simulink model "Scheme"  (R2014a)
settings: Solver=ode45  SolverMode=SingleTasking  StartTime=0.0  StopTime=5.0  RelTol=1e-3
libraries: commsink2 x1, dspsigops x1, simulink x1, dspsrcs4 x1
settings Model: Creator=Olia  LastModifiedBy=olia-PC
settings OptimizationCC: BlockReduction=off  BooleanDataType=off  SimCompilerOptimization=off
settings DebuggingCC: SaveWithParameterizedLinksMsg=none  UnderspecifiedInitializationDetection=Classic  SignalResolutionControl=TryResolveAllWithWarning  SolverPrmCheckMsg=none  FrameProcessingCompatibilityMsg=error  StrictBusMsg=Warning
settings HardwareCC: TargetUnknown=on
settings RTWCC: RTWCompilerOptimization=off

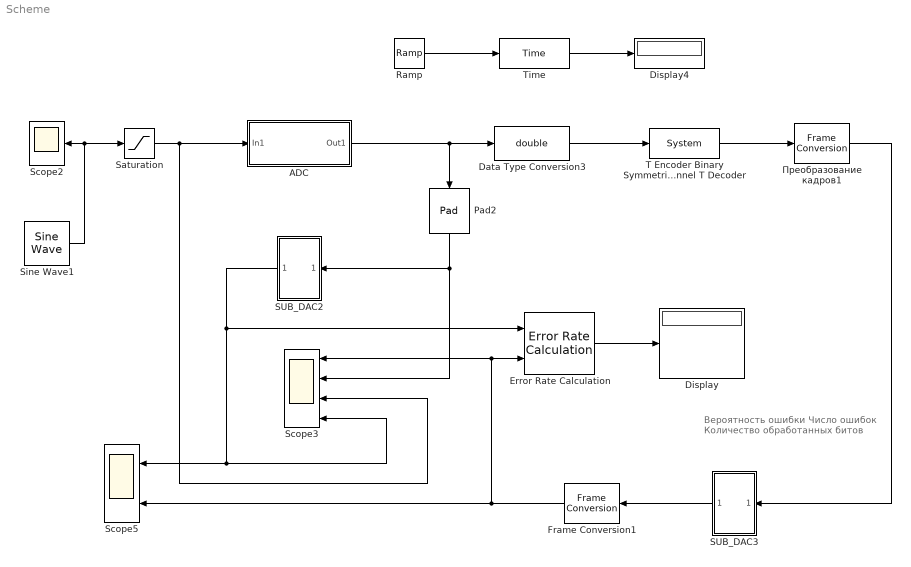
== system Scheme ==
  note: Вероятность ошибки
      | Число ошибок
      | Количество обработанных битов
  ADC : Subsystem
  Data Type Conversion3 : DataTypeConversion  OutDataTypeStr=double
  Display : Display
  Display4 : Display
  Error Rate Calculation : commsink2/Error Rate Calculation  N=0  st_delay=0  cp_mode=Entire frame  subframe=[]  PMode=Port  WsName=ErrorVec1  RsMode2=off  stop=off  numErr=maxNumErrs  maxBits=maxNumBits
  Frame Conversion1 : FrameConversion  OutFrame=Sample-based
  Pad2 : dspsigops/Pad  padAlong=Columns  dimsToPad=1  valSrc=Specify via dialog  padVal=1  spec=Output size  padNumOutRowsSpecMethod=User-specified  numOutRows=16  padNumOutColsSpecMethod=User-specified  numOutCols=1  isVarDimsMode=off  padBeginning=0  padEnd=0  outSizeMode=User-specified  outSize=1  padSigAt=Beginning  trunc_flag=None  roundingMode=Floor  overflowMode=off  truncOrWrapMode=Truncate  wrap_flag=None
  Ramp : simulink/Sources/Ramp  slope=1  start=0  X0=0
  SUB_DAC2 : Subsystem
  SUB_DAC3 : Subsystem
  Saturation : Saturate  UpperLimit=2^24-1  LowerLimit=0
  Scope2 : Scope
      settings: TickLabels=on  YMin=0  YMax=10  SaveName=ScopeData2
  Scope3 : Scope  NumInputPorts=4
      settings: TickLabels=on  TimeRange=3  YMin=0~-5~-5~-5  YMax=3~10~10~5  SaveName=ScopeData5
  Scope5 : Scope  NumInputPorts=2
      settings: TickLabels=on  YMin=0~0  YMax=3~6e-06  SaveName=ScopeData4
  Sine Wave1 : dspsrcs4/Sine Wave  Amplitude=10  Frequency=2  Phase=0  SampleMode=Discrete  OutComplex=Real  CompMethod=Trigonometric fcn  TableSize=Speed  SampleTime=1/70  SamplesPerFrame=1  ResetState=Restart at time zero  dataType=double  wordLen=16  udDataType=sfix(16)  fracBitsMode=Best precision  numFracBits=15  OutDataTypeStr=double  LastOutDataTypeStr=double
  T Encoder Binary Symmetric Channel T Decoder : MATLABFcn  MATLABFcn=System
  Time : MATLABFcn  MATLABFcn=Time
  Преобразование кадров1 : FrameConversion
  wires:
  Error Rate Calculation/1 -> Display/1
  Sine Wave1/1 -> Scope2/1, Saturation/1
  Saturation/1 -> Scope3/3, ADC/1(In1)
  SUB_DAC3/1(Out1) -> Frame Conversion1/1
  Frame Conversion1/1 -> Scope5/2, Scope3/1, Error Rate Calculation/2
  SUB_DAC2/1(Out1) -> Scope3/4, Scope5/1, Error Rate Calculation/1
  ADC/1(Out1) -> Pad2/1, Data Type Conversion3/1
  Преобразование кадров1/1 -> SUB_DAC3/1(In2)
  Pad2/1 -> Scope3/2, SUB_DAC2/1(In2)
  Time/1 -> Display4/1
  Ramp/1 -> Time/1
  Data Type Conversion3/1 -> T Encoder Binary Symmetric Channel T Decoder/1
  T Encoder Binary Symmetric Channel T Decoder/1 -> Преобразование кадров1/1

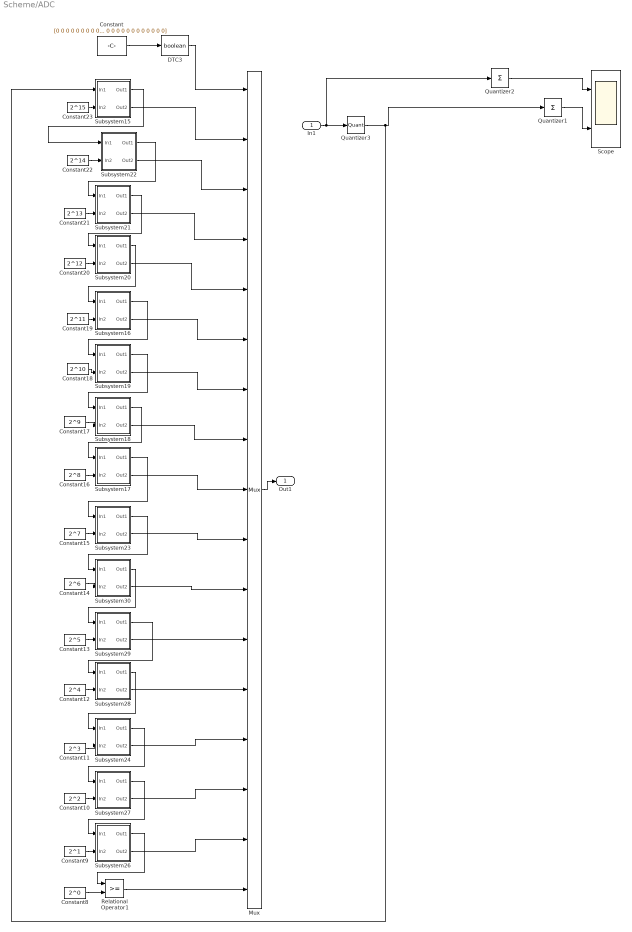
== system Scheme/ADC ==
  In1 : Inport
  Constant : Constant  Value=[0 0 0 0 0 0 0 0 0 0 0 0 0 0 0 0 0 0 0 0 0 0 0 0 0 0 0 0 0 0 0 0 0 0 0 0 0 0 0 0 0 0 0 0 0 0 0 0 0 0 0 0 0 0 0]
  Constant10 : Constant  Value=2^2
  Constant11 : Constant  Value=2^3
  Constant12 : Constant  Value=2^4
  Constant13 : Constant  Value=2^5
  Constant14 : Constant  Value=2^6
  Constant15 : Constant  Value=2^7
  Constant16 : Constant  Value=2^8
  Constant17 : Constant  Value=2^9
  Constant18 : Constant  Value=2^10
  Constant19 : Constant  Value=2^11
  Constant20 : Constant  Value=2^12
  Constant21 : Constant  Value=2^13
  Constant22 : Constant  Value=2^14
  Constant23 : Constant  Value=2^15
  Constant8 : Constant  Value=2^0
  Constant9 : Constant  Value=2^1
  DTC3 : DataTypeConversion  OutDataTypeStr=boolean  LockScale=on
  Mux : Mux  Inputs=17
  Quantizer1 : Sum  Inputs=+
  Quantizer2 : Sum  Inputs=+
  Quantizer3 : Quantizer  QuantizationInterval=0.2
  Relational Operator1 : RelationalOperator  OutDataTypeStr=boolean
  Scope : Scope  NumInputPorts=2
      settings: YMin=-5~-5  YMax=5~5
  Subsystem15 : Subsystem
  Subsystem16 : Subsystem
  Subsystem17 : Subsystem
  Subsystem18 : Subsystem
  Subsystem19 : Subsystem
  Subsystem20 : Subsystem
  Subsystem21 : Subsystem
  Subsystem22 : Subsystem
  Subsystem23 : Subsystem
  Subsystem24 : Subsystem
  Subsystem26 : Subsystem
  Subsystem27 : Subsystem
  Subsystem28 : Subsystem
  Subsystem29 : Subsystem
  Subsystem30 : Subsystem
  Out1 : Outport
  wires:
  Subsystem15/1(Out1) -> Subsystem22/1(In1)
  Quantizer3/1 -> Quantizer1/1, Subsystem15/1(In1)
  Quantizer1/1 -> Scope/2
  Quantizer2/1 -> Scope/1
  Mux/1 -> Out1/1
  In1/1 -> Quantizer2/1, Quantizer3/1
  Subsystem28/1(Out1) -> Subsystem24/1(In1)
  Constant11/1 -> Subsystem24/2(In2)
  Subsystem20/1(Out1) -> Subsystem16/1(In1)
  Subsystem17/1(Out1) -> Subsystem23/1(In1)
  Subsystem26/1(Out1) -> Relational Operator1/1
  Subsystem29/1(Out1) -> Subsystem28/1(In1)
  Subsystem18/1(Out1) -> Subsystem17/1(In1)
  Subsystem21/1(Out1) -> Subsystem20/1(In1)
  Constant22/1 -> Subsystem22/2(In2)
  Constant21/1 -> Subsystem21/2(In2)
  Constant19/1 -> Subsystem16/2(In2)
  Constant20/1 -> Subsystem20/2(In2)
  Constant9/1 -> Subsystem26/2(In2)
  Constant10/1 -> Subsystem27/2(In2)
  Constant12/1 -> Subsystem28/2(In2)
  Constant13/1 -> Subsystem29/2(In2)
  Constant14/1 -> Subsystem30/2(In2)
  Constant15/1 -> Subsystem23/2(In2)
  Constant16/1 -> Subsystem17/2(In2)
  Constant17/1 -> Subsystem18/2(In2)
  Constant18/1 -> Subsystem19/2(In2)
  Constant23/1 -> Subsystem15/2(In2)
  Constant8/1 -> Relational Operator1/2
  Subsystem27/1(Out1) -> Subsystem26/1(In1)
  Subsystem24/1(Out1) -> Subsystem27/1(In1)
  Subsystem30/1(Out1) -> Subsystem29/1(In1)
  Subsystem23/1(Out1) -> Subsystem30/1(In1)
  Subsystem19/1(Out1) -> Subsystem18/1(In1)
  Subsystem16/1(Out1) -> Subsystem19/1(In1)
  Subsystem22/1(Out1) -> Subsystem21/1(In1)
  Relational Operator1/1 -> Mux/17
  Subsystem26/2(Out2) -> Mux/16
  Subsystem27/2(Out2) -> Mux/15
  Subsystem24/2(Out2) -> Mux/14
  Subsystem28/2(Out2) -> Mux/13
  Subsystem29/2(Out2) -> Mux/12
  Subsystem30/2(Out2) -> Mux/11
  Subsystem23/2(Out2) -> Mux/10
  Subsystem17/2(Out2) -> Mux/9
  Subsystem18/2(Out2) -> Mux/8
  Subsystem19/2(Out2) -> Mux/7
  Subsystem16/2(Out2) -> Mux/6
  Subsystem20/2(Out2) -> Mux/5
  Subsystem21/2(Out2) -> Mux/4
  Subsystem22/2(Out2) -> Mux/3
  Subsystem15/2(Out2) -> Mux/2
  Constant/1 -> DTC3/1
  DTC3/1 -> Mux/1

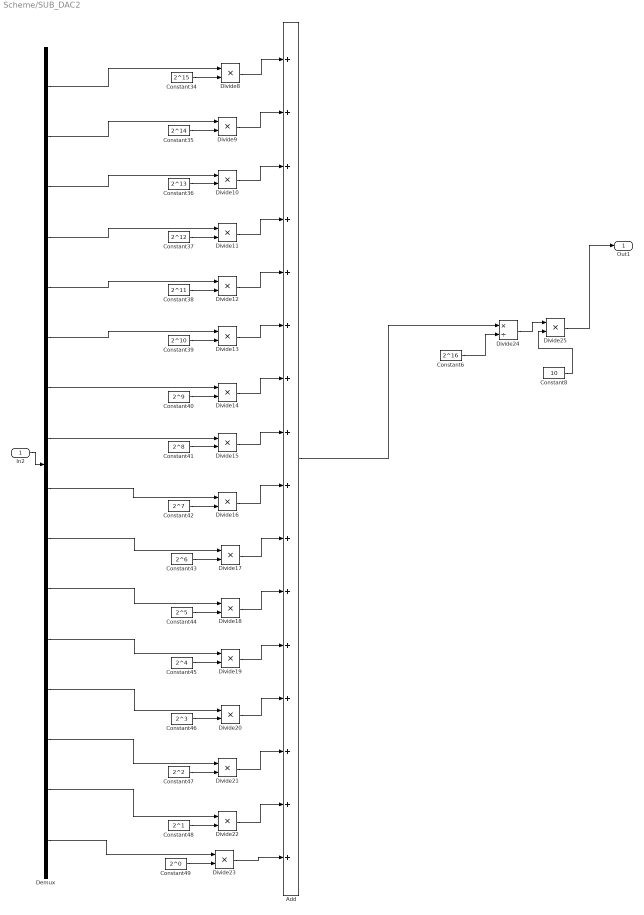
== system Scheme/SUB_DAC2 ==
  In2 : Inport
  Add : Sum  Inputs=++++++++++++++++
  Constant34 : Constant  Value=2^15
  Constant35 : Constant  Value=2^14
  Constant36 : Constant  Value=2^13
  Constant37 : Constant  Value=2^12
  Constant38 : Constant  Value=2^11
  Constant39 : Constant  Value=2^10
  Constant40 : Constant  Value=2^9
  Constant41 : Constant  Value=2^8
  Constant42 : Constant  Value=2^7
  Constant43 : Constant  Value=2^6
  Constant44 : Constant  Value=2^5
  Constant45 : Constant  Value=2^4
  Constant46 : Constant  Value=2^3
  Constant47 : Constant  Value=2^2
  Constant48 : Constant  Value=2^1
  Constant49 : Constant  Value=2^0
  Constant6 : Constant  Value=2^16
  Constant8 : Constant  Value=10
  Demux : Demux  Outputs=16
  Divide{8..23,25} (17 alike) : Product  Inputs=**
  Divide24 : Product  Inputs=*/
  Out1 : Outport
  wires:
  Constant49/1 -> Divide23/2
  Constant48/1 -> Divide22/2
  Constant47/1 -> Divide21/2
  Constant46/1 -> Divide20/2
  Constant45/1 -> Divide19/2
  Constant44/1 -> Divide18/2
  Constant43/1 -> Divide17/2
  Constant42/1 -> Divide16/2
  Constant41/1 -> Divide15/2
  Constant40/1 -> Divide14/2
  Constant39/1 -> Divide13/2
  Constant38/1 -> Divide12/2
  Constant37/1 -> Divide11/2
  Constant36/1 -> Divide10/2
  Constant35/1 -> Divide9/2
  Constant34/1 -> Divide8/2
  In2/1 -> Demux/1
  Add/1 -> Divide24/1
  Constant6/1 -> Divide24/2
  Divide24/1 -> Divide25/1
  Constant8/1 -> Divide25/2
  Divide25/1 -> Out1/1
  Divide23/1 -> Add/16
  Divide22/1 -> Add/15
  Divide21/1 -> Add/14
  Divide20/1 -> Add/13
  Divide19/1 -> Add/12
  Divide18/1 -> Add/11
  Divide17/1 -> Add/10
  Divide16/1 -> Add/9
  Divide15/1 -> Add/8
  Divide14/1 -> Add/7
  Divide13/1 -> Add/6
  Divide12/1 -> Add/5
  Divide11/1 -> Add/4
  Divide10/1 -> Add/3
  Divide9/1 -> Add/2
  Divide8/1 -> Add/1
  Demux/1 -> Divide8/1
  Demux/2 -> Divide9/1
  Demux/3 -> Divide10/1
  Demux/4 -> Divide11/1
  Demux/5 -> Divide12/1
  Demux/6 -> Divide13/1
  Demux/7 -> Divide14/1
  Demux/8 -> Divide15/1
  Demux/9 -> Divide16/1
  Demux/10 -> Divide17/1
  Demux/11 -> Divide18/1
  Demux/12 -> Divide19/1
  Demux/13 -> Divide20/1
  Demux/14 -> Divide21/1
  Demux/15 -> Divide22/1
  Demux/16 -> Divide23/1

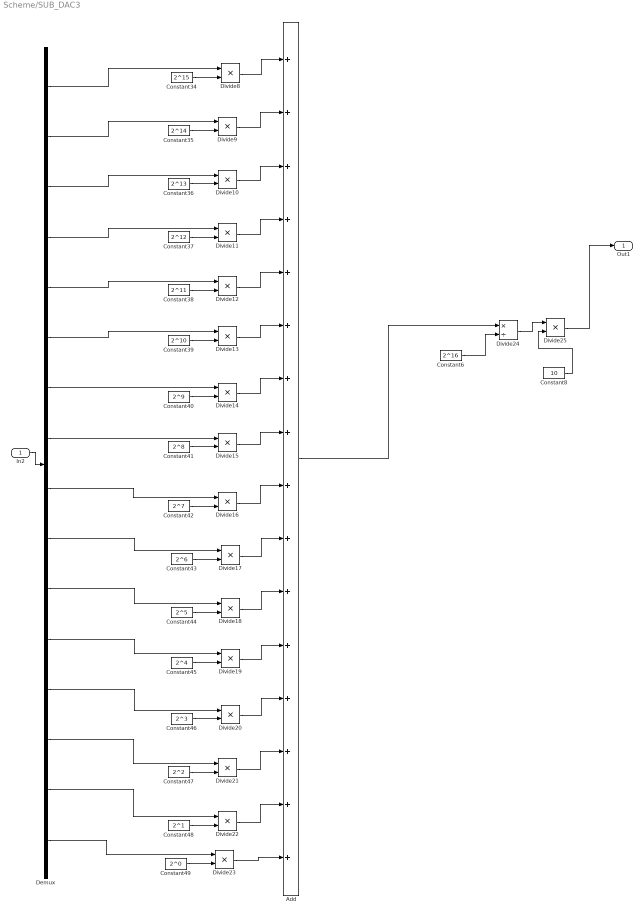
== system Scheme/SUB_DAC3 ==
  In2 : Inport
  Add : Sum  Inputs=++++++++++++++++
  Constant34 : Constant  Value=2^15
  Constant35 : Constant  Value=2^14
  Constant36 : Constant  Value=2^13
  Constant37 : Constant  Value=2^12
  Constant38 : Constant  Value=2^11
  Constant39 : Constant  Value=2^10
  Constant40 : Constant  Value=2^9
  Constant41 : Constant  Value=2^8
  Constant42 : Constant  Value=2^7
  Constant43 : Constant  Value=2^6
  Constant44 : Constant  Value=2^5
  Constant45 : Constant  Value=2^4
  Constant46 : Constant  Value=2^3
  Constant47 : Constant  Value=2^2
  Constant48 : Constant  Value=2^1
  Constant49 : Constant  Value=2^0
  Constant6 : Constant  Value=2^16
  Constant8 : Constant  Value=10
  Demux : Demux  Outputs=16
  Divide{8..23,25} (17 alike) : Product  Inputs=**
  Divide24 : Product  Inputs=*/
  Out1 : Outport
  wires:
  Demux/16 -> Divide23/1
  Demux/15 -> Divide22/1
  Demux/14 -> Divide21/1
  Demux/13 -> Divide20/1
  Demux/12 -> Divide19/1
  Demux/11 -> Divide18/1
  Demux/10 -> Divide17/1
  Demux/9 -> Divide16/1
  Demux/8 -> Divide15/1
  Demux/7 -> Divide14/1
  Demux/6 -> Divide13/1
  Demux/5 -> Divide12/1
  Demux/4 -> Divide11/1
  Demux/3 -> Divide10/1
  Demux/2 -> Divide9/1
  Demux/1 -> Divide8/1
  Divide8/1 -> Add/1
  Divide9/1 -> Add/2
  Divide10/1 -> Add/3
  Divide11/1 -> Add/4
  Divide12/1 -> Add/5
  Divide13/1 -> Add/6
  Divide14/1 -> Add/7
  Divide15/1 -> Add/8
  Divide16/1 -> Add/9
  Divide17/1 -> Add/10
  Divide18/1 -> Add/11
  Divide19/1 -> Add/12
  Divide20/1 -> Add/13
  Divide21/1 -> Add/14
  Divide22/1 -> Add/15
  Divide23/1 -> Add/16
  Divide25/1 -> Out1/1
  Constant8/1 -> Divide25/2
  Divide24/1 -> Divide25/1
  Constant6/1 -> Divide24/2
  Add/1 -> Divide24/1
  In2/1 -> Demux/1
  Constant34/1 -> Divide8/2
  Constant35/1 -> Divide9/2
  Constant36/1 -> Divide10/2
  Constant37/1 -> Divide11/2
  Constant38/1 -> Divide12/2
  Constant39/1 -> Divide13/2
  Constant40/1 -> Divide14/2
  Constant41/1 -> Divide15/2
  Constant42/1 -> Divide16/2
  Constant43/1 -> Divide17/2
  Constant44/1 -> Divide18/2
  Constant45/1 -> Divide19/2
  Constant46/1 -> Divide20/2
  Constant47/1 -> Divide21/2
  Constant48/1 -> Divide22/2
  Constant49/1 -> Divide23/2

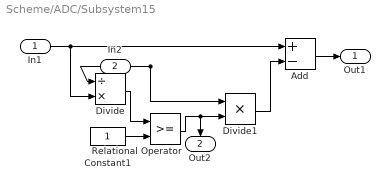
== system Scheme/ADC/Subsystem15 ==
  In1 : Inport
  In2 : Inport  Port=2
  Add : Sum  Inputs=+-
  Constant1 : Constant
  Divide : Product  Inputs=/*
  Divide1 : Product  Inputs=**
  Relational Operator : RelationalOperator  OutDataTypeStr=boolean
  Out1 : Outport
  Out2 : Outport  Port=2
  wires:
  Divide/1 -> Relational Operator/1
  Constant1/1 -> Relational Operator/2
  Relational Operator/1 -> Divide1/2, Out2/1
  Divide1/1 -> Add/2
  In2/1 -> Divide/1, Divide1/1
  In1/1 -> Divide/2, Add/1
  Add/1 -> Out1/1

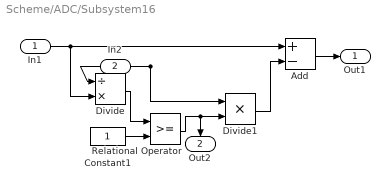
== system Scheme/ADC/Subsystem16 ==
  In1 : Inport
  In2 : Inport  Port=2
  Add : Sum  Inputs=+-
  Constant1 : Constant
  Divide : Product  Inputs=/*
  Divide1 : Product  Inputs=**
  Relational Operator : RelationalOperator  OutDataTypeStr=boolean
  Out1 : Outport
  Out2 : Outport  Port=2
  wires:
  Add/1 -> Out1/1
  In1/1 -> Add/1, Divide/2
  In2/1 -> Divide1/1, Divide/1
  Divide1/1 -> Add/2
  Relational Operator/1 -> Out2/1, Divide1/2
  Constant1/1 -> Relational Operator/2
  Divide/1 -> Relational Operator/1

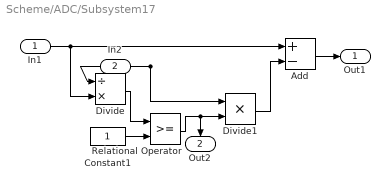
== system Scheme/ADC/Subsystem17 ==
  In1 : Inport
  In2 : Inport  Port=2
  Add : Sum  Inputs=+-
  Constant1 : Constant
  Divide : Product  Inputs=/*
  Divide1 : Product  Inputs=**
  Relational Operator : RelationalOperator  OutDataTypeStr=boolean
  Out1 : Outport
  Out2 : Outport  Port=2
  wires:
  Divide/1 -> Relational Operator/1
  Constant1/1 -> Relational Operator/2
  Relational Operator/1 -> Divide1/2, Out2/1
  Divide1/1 -> Add/2
  In2/1 -> Divide/1, Divide1/1
  In1/1 -> Divide/2, Add/1
  Add/1 -> Out1/1

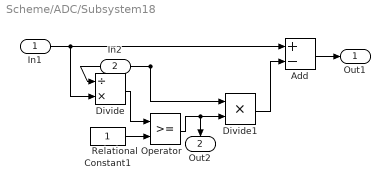
== system Scheme/ADC/Subsystem18 ==
  In1 : Inport
  In2 : Inport  Port=2
  Add : Sum  Inputs=+-
  Constant1 : Constant
  Divide : Product  Inputs=/*
  Divide1 : Product  Inputs=**
  Relational Operator : RelationalOperator  OutDataTypeStr=boolean
  Out1 : Outport
  Out2 : Outport  Port=2
  wires:
  Add/1 -> Out1/1
  In1/1 -> Add/1, Divide/2
  In2/1 -> Divide1/1, Divide/1
  Divide1/1 -> Add/2
  Relational Operator/1 -> Out2/1, Divide1/2
  Constant1/1 -> Relational Operator/2
  Divide/1 -> Relational Operator/1

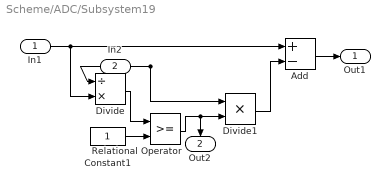
== system Scheme/ADC/Subsystem19 ==
  In1 : Inport
  In2 : Inport  Port=2
  Add : Sum  Inputs=+-
  Constant1 : Constant
  Divide : Product  Inputs=/*
  Divide1 : Product  Inputs=**
  Relational Operator : RelationalOperator  OutDataTypeStr=boolean
  Out1 : Outport
  Out2 : Outport  Port=2
  wires:
  Divide/1 -> Relational Operator/1
  Constant1/1 -> Relational Operator/2
  Relational Operator/1 -> Divide1/2, Out2/1
  Divide1/1 -> Add/2
  In2/1 -> Divide/1, Divide1/1
  In1/1 -> Divide/2, Add/1
  Add/1 -> Out1/1

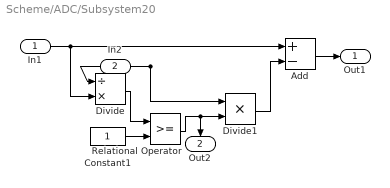
== system Scheme/ADC/Subsystem20 ==
  In1 : Inport
  In2 : Inport  Port=2
  Add : Sum  Inputs=+-
  Constant1 : Constant
  Divide : Product  Inputs=/*
  Divide1 : Product  Inputs=**
  Relational Operator : RelationalOperator  OutDataTypeStr=boolean
  Out1 : Outport
  Out2 : Outport  Port=2
  wires:
  Add/1 -> Out1/1
  In1/1 -> Add/1, Divide/2
  In2/1 -> Divide1/1, Divide/1
  Divide1/1 -> Add/2
  Relational Operator/1 -> Out2/1, Divide1/2
  Constant1/1 -> Relational Operator/2
  Divide/1 -> Relational Operator/1

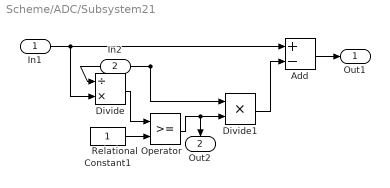
== system Scheme/ADC/Subsystem21 ==
  In1 : Inport
  In2 : Inport  Port=2
  Add : Sum  Inputs=+-
  Constant1 : Constant
  Divide : Product  Inputs=/*
  Divide1 : Product  Inputs=**
  Relational Operator : RelationalOperator  OutDataTypeStr=boolean
  Out1 : Outport
  Out2 : Outport  Port=2
  wires:
  Divide/1 -> Relational Operator/1
  Constant1/1 -> Relational Operator/2
  Relational Operator/1 -> Divide1/2, Out2/1
  Divide1/1 -> Add/2
  In2/1 -> Divide/1, Divide1/1
  In1/1 -> Divide/2, Add/1
  Add/1 -> Out1/1

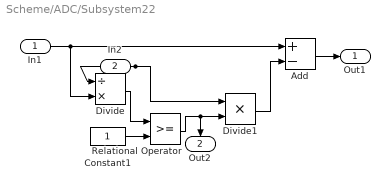
== system Scheme/ADC/Subsystem22 ==
  In1 : Inport
  In2 : Inport  Port=2
  Add : Sum  Inputs=+-
  Constant1 : Constant
  Divide : Product  Inputs=/*
  Divide1 : Product  Inputs=**
  Relational Operator : RelationalOperator  OutDataTypeStr=boolean
  Out1 : Outport
  Out2 : Outport  Port=2
  wires:
  Add/1 -> Out1/1
  In1/1 -> Add/1, Divide/2
  In2/1 -> Divide1/1, Divide/1
  Divide1/1 -> Add/2
  Relational Operator/1 -> Out2/1, Divide1/2
  Constant1/1 -> Relational Operator/2
  Divide/1 -> Relational Operator/1

== system Scheme/ADC/Subsystem23 ==
  In1 : Inport
  In2 : Inport  Port=2
  Add : Sum  Inputs=+-
  Constant1 : Constant
  Divide : Product  Inputs=/*
  Divide1 : Product  Inputs=**
  Relational Operator : RelationalOperator  OutDataTypeStr=boolean
  Out1 : Outport
  Out2 : Outport  Port=2
  wires:
  Add/1 -> Out1/1
  In1/1 -> Add/1, Divide/2
  In2/1 -> Divide1/1, Divide/1
  Divide1/1 -> Add/2
  Relational Operator/1 -> Out2/1, Divide1/2
  Constant1/1 -> Relational Operator/2
  Divide/1 -> Relational Operator/1

== system Scheme/ADC/Subsystem24 ==
  In1 : Inport
  In2 : Inport  Port=2
  Add : Sum  Inputs=+-
  Constant1 : Constant
  Divide : Product  Inputs=/*
  Divide1 : Product  Inputs=**
  Relational Operator : RelationalOperator  OutDataTypeStr=boolean
  Out1 : Outport
  Out2 : Outport  Port=2
  wires:
  Divide/1 -> Relational Operator/1
  Constant1/1 -> Relational Operator/2
  Relational Operator/1 -> Divide1/2, Out2/1
  Divide1/1 -> Add/2
  In2/1 -> Divide/1, Divide1/1
  In1/1 -> Divide/2, Add/1
  Add/1 -> Out1/1

== system Scheme/ADC/Subsystem26 ==
  In1 : Inport
  In2 : Inport  Port=2
  Add : Sum  Inputs=+-
  Constant1 : Constant
  Divide : Product  Inputs=/*
  Divide1 : Product  Inputs=**
  Relational Operator : RelationalOperator  OutDataTypeStr=boolean
  Out1 : Outport
  Out2 : Outport  Port=2
  wires:
  Divide/1 -> Relational Operator/1
  Constant1/1 -> Relational Operator/2
  Relational Operator/1 -> Divide1/2, Out2/1
  Divide1/1 -> Add/2
  In2/1 -> Divide/1, Divide1/1
  In1/1 -> Divide/2, Add/1
  Add/1 -> Out1/1

== system Scheme/ADC/Subsystem27 ==
  In1 : Inport
  In2 : Inport  Port=2
  Add : Sum  Inputs=+-
  Constant1 : Constant
  Divide : Product  Inputs=/*
  Divide1 : Product  Inputs=**
  Relational Operator : RelationalOperator  OutDataTypeStr=boolean
  Out1 : Outport
  Out2 : Outport  Port=2
  wires:
  Add/1 -> Out1/1
  In1/1 -> Add/1, Divide/2
  In2/1 -> Divide1/1, Divide/1
  Divide1/1 -> Add/2
  Relational Operator/1 -> Out2/1, Divide1/2
  Constant1/1 -> Relational Operator/2
  Divide/1 -> Relational Operator/1

== system Scheme/ADC/Subsystem28 ==
  In1 : Inport
  In2 : Inport  Port=2
  Add : Sum  Inputs=+-
  Constant1 : Constant
  Divide : Product  Inputs=/*
  Divide1 : Product  Inputs=**
  Relational Operator : RelationalOperator  OutDataTypeStr=boolean
  Out1 : Outport
  Out2 : Outport  Port=2
  wires:
  Divide/1 -> Relational Operator/1
  Constant1/1 -> Relational Operator/2
  Relational Operator/1 -> Divide1/2, Out2/1
  Divide1/1 -> Add/2
  In2/1 -> Divide/1, Divide1/1
  In1/1 -> Divide/2, Add/1
  Add/1 -> Out1/1

== system Scheme/ADC/Subsystem29 ==
  In1 : Inport
  In2 : Inport  Port=2
  Add : Sum  Inputs=+-
  Constant1 : Constant
  Divide : Product  Inputs=/*
  Divide1 : Product  Inputs=**
  Relational Operator : RelationalOperator  OutDataTypeStr=boolean
  Out1 : Outport
  Out2 : Outport  Port=2
  wires:
  Add/1 -> Out1/1
  In1/1 -> Add/1, Divide/2
  In2/1 -> Divide1/1, Divide/1
  Divide1/1 -> Add/2
  Relational Operator/1 -> Out2/1, Divide1/2
  Constant1/1 -> Relational Operator/2
  Divide/1 -> Relational Operator/1

== system Scheme/ADC/Subsystem30 ==
  In1 : Inport
  In2 : Inport  Port=2
  Add : Sum  Inputs=+-
  Constant1 : Constant
  Divide : Product  Inputs=/*
  Divide1 : Product  Inputs=**
  Relational Operator : RelationalOperator  OutDataTypeStr=boolean
  Out1 : Outport
  Out2 : Outport  Port=2
  wires:
  Divide/1 -> Relational Operator/1
  Constant1/1 -> Relational Operator/2
  Relational Operator/1 -> Divide1/2, Out2/1
  Divide1/1 -> Add/2
  In2/1 -> Divide/1, Divide1/1
  In1/1 -> Divide/2, Add/1
  Add/1 -> Out1/1
